simulink model "zodModel"  (R2014b)
settings: Solver=ode45  StartTime=0.0  StopTime=145*T  FixedStep=T  MaxStep=T  RelTol=1e-3
StopFcn:
  | save(wSaveFileName,wSaveFileName)
values from neighbouring files (symbols this model uses):
  wContinuousSystemDen = [1,11,30,200]    [ZTransformDataDictionnary.m]
  wContinuousSystemNum = 100    [ZTransformDataDictionnary.m]
undefined symbols (not defined in the file or in its folder): Hbox, T, wYboxD, wYhalD, wYhalN, wYtutD, wYtutN, wYzodD, wYzodN
settings Model: Creator=Zangdaarr  LastModifiedBy=Zangdaarr

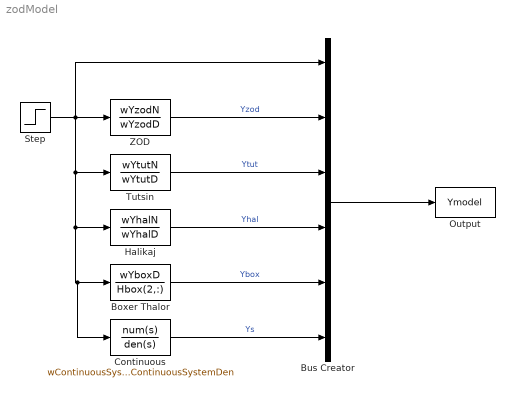
== system zodModel ==
  Boxer Thalor : DiscreteTransferFcn  Numerator=wYboxD  Denominator=Hbox(2,:)  SampleTime=T
  Bus Creator : BusCreator  Inputs=6
  Continuous : TransferFcn  Numerator=wContinuousSystemNum  Denominator=wContinuousSystemDen
  Halikaj : DiscreteTransferFcn  Numerator=wYhalN  Denominator=wYhalD  SampleTime=T
  Output : ToWorkspace  VariableName=Ymodel  SaveFormat=Timeseries  SampleTime=-1
  Step : Step  Time=0  SampleTime=0
  Tutsin : DiscreteTransferFcn  Numerator=wYtutN  Denominator=wYtutD  SampleTime=T
  ZOD : DiscreteTransferFcn  Numerator=wYzodN  Denominator=wYzodD  SampleTime=T
  wires:
  Step/1 -> Halikaj/1, Continuous/1, Boxer Thalor/1, Tutsin/1, Bus Creator/1, ZOD/1
  ZOD/1 -> Bus Creator/2  "Yzod"
  Tutsin/1 -> Bus Creator/3  "Ytut"
  Bus Creator/1 -> Output/1
  Boxer Thalor/1 -> Bus Creator/5  "Ybox"
  Halikaj/1 -> Bus Creator/4  "Yhal"
  Continuous/1 -> Bus Creator/6  "Ys"
